simulink model "TestGammaVar"  (R2015a)
settings: Solver=ode45  StartTime=0.0  StopTime=10.0  RelTol=1e-3
values from neighbouring files (symbols this model uses):
  A1 = 254.469    [LQG_LTR_fen.m]    (also in LQG_LTR_ident.m = 245; LQG_LTR_pheno.m)
  A2 = 254.469    [LQG_LTR_fen.m]    (also in LQG_LTR_ident.m = 270; LQG_LTR_pheno.m)
  A3 = 254.469    [LQG_LTR_fen.m]    (also in LQG_LTR_ident.m; LQG_LTR_pheno.m)
  A4 = 254.469    [LQG_LTR_fen.m]    (also in LQG_LTR_ident.m; LQG_LTR_pheno.m)
  k1 = 18    [LQG_LTR_fen.m]    (also in LQG_LTR_ident.m; LQG_LTR_pheno.m = 12)
  k2 = 18    [LQG_LTR_fen.m]    (also in LQG_LTR_ident.m; LQG_LTR_pheno.m = 12)
settings Model: Creator=plinio  LastModifiedBy=plinio

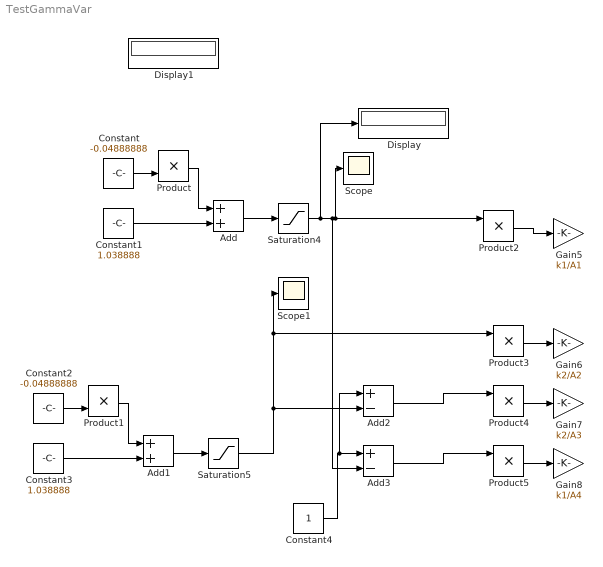
== system TestGammaVar ==
  Add : Sum
  Add1 : Sum
  Add2 : Sum  Inputs=+-
  Add3 : Sum  Inputs=+-
  Constant : Constant  Value=-0.04888888
  Constant1 : Constant  Value=1.038888
  Constant2 : Constant  Value=-0.04888888
  Constant3 : Constant  Value=1.038888
  Constant4 : Constant
  Display : Display
  Display1 : Display
  Gain5 : Gain  Gain=k1/A1
  Gain6 : Gain  Gain=k2/A2
  Gain7 : Gain  Gain=k2/A3
  Gain8 : Gain  Gain=k1/A4
  Product{,1..5} (6 alike) : Product
  Saturation4 : Saturate  UpperLimit=1  LowerLimit=0.55
  Saturation5 : Saturate  UpperLimit=1  LowerLimit=0.55
  Scope : Scope
      settings: SaveName=ScopeData4
  Scope1 : Scope
      settings: SaveName=ScopeData5
  wires:
  Constant1/1 -> Add/2
  Constant/1 -> Product/2
  Product/1 -> Add/1
  Add/1 -> Saturation4/1
  Saturation4/1 -> Display/1, Product2/1, Scope/1, Add3/2
  Constant3/1 -> Add1/2
  Constant2/1 -> Product1/2
  Product1/1 -> Add1/1
  Add1/1 -> Saturation5/1
  ? -> Product1/1, Product4/2, Product3/2
  Constant4/1 -> Add2/1, Add3/1
  Saturation5/1 -> Add2/2, Product3/1, Scope1/1
  ? -> Product5/2, Product2/2, Display1/1, Product/1
  Product2/1 -> Gain5/1
  Product3/1 -> Gain6/1
  Product4/1 -> Gain7/1
  Product5/1 -> Gain8/1
  Add2/1 -> Product4/1
  Add3/1 -> Product5/1
